simulink model "modelo_XP_LQRY_GUIA"  (R2025b)
settings: Solver=ode4  StartTime=0.0  StopTime=TimeXP  FixedStep=Ts  RelTol=1e-3
values from neighbouring files (symbols this model uses):
  att_alt = 0    [XP_doublets_lqry2.m]    (also in XP_missao_lqry.m; XP_missao_lqry2.m)
  h_ref0 = h_ref    [NL_missao.m]    (also in XP_doublets_lqry2.m = 600; XP_missao.m; XP_missao_lqry.m = XP_h_ref0; XP_missao_lqry2.m = XP_h_ref0)
  phi_psi = XP_dbl_phi_psi    [XP_doublets_lqry2.m]    (also in XP_missao_lqry.m = 0; XP_missao_lqry2.m = cfg_user.phipsi)
  R_accept = cfgm.R    [NL_missao.m]    (also in XP_doublets_lqry2.m = 80; XP_missao.m = XP_R_accept; XP_missao_lqry.m = cfg_user.R; XP_missao_lqry2.m = cfg_user.R)
  refAlt = XP_dbl_refAlt    [XP_doublets_lqry2.m]    (also in XP_missao_lqry.m = 0; XP_missao_lqry2.m = 0)
  refPhi = XP_dbl_refPhi    [XP_doublets_lqry2.m]    (also in XP_missao_lqry.m = 0; XP_missao_lqry2.m = 0)
  refPsi = XP_dbl_refPsi    [XP_doublets_lqry2.m]    (also in XP_missao_lqry.m = 0; XP_missao_lqry2.m = 0)
  reftheta = 0    [XP_doublets_lqry2.m]    (also in XP_missao_lqry.m; XP_missao_lqry2.m)
  refVel = XP_dbl_VT    [XP_doublets_lqry2.m]    (also in XP_missao_lqry.m = 12; XP_missao_lqry2.m = 12)
  VT_ref0 = VT_ref    [NL_missao.m]    (also in XP_doublets_lqry2.m = XP_dbl_VT; XP_missao.m; XP_missao_lqry.m = 12; XP_missao_lqry2.m = 12)
  VT_Throttle = XP_dbl_VT_Throttle    [XP_doublets_lqry2.m]    (also in XP_missao_lqry.m = 1; XP_missao_lqry2.m = 1)
  WPs = WPs_user(1,:)    [NL_missao.m]    (also in XP_doublets_lqry2.m = WPs_user; WPs(:,1:2) = ne'; XP_missao.m; XP_missao_lqry.m; XP_missao_lqry2.m)
  Xe = montaX(y)    [VR_plot_sato_real.m]    (also in VR_tic.m; plot_degrau_3vias_sato.m)
  XP_h_ref0 = XP_msl0    (= 600)    [XP_doublets_lqry2.m]    (also in XP_missao_lqry.m = XP_msl0; XP_missao_lqry2.m = XP_msl0)
  XP_IC_int_alt = double((0 - GsA*[x4_dev; 0]) / GiA)    [XP_doublets_lqry2.m]    (also in XP_missao_lqry.m = (theta0 - GstateLong_Alt*[x4; 0]) / GintLong_Alt; XP_missao_lqry2.m = double((theta0 - GsA*[x4; 0]) / GiA))
  XP_IC_int_speed = double((thr_delta0*100 - GsS*x4_dev) / GiS)    [XP_doublets_lqry2.m]    (also in XP_missao_lqry.m = (XP_thr0*100 - GstateLong_speed*x4) / GintLong_speed; XP_missao_lqry2.m = double((thr_delta0*100 - GsS*x4) / GiS))
  XP_IC_int_theta = double((de_delta0*(1 - GsT(5)) - GsT(1:4)*x4_dev) / GiT)    [XP_doublets_lqry2.m]    (also in XP_missao_lqry.m = (XP_de0_dg*(1 - GstateLong(5)) - GstateLong(1:4)*x4) / GintL; XP_missao_lqry2.m = double((de_delta0*(1 - GsT(5)) - GsT(1:4)*x4) / GiT))
undefined symbols (not defined in the file or in its folder): Gintlat, Gintlat_psi, GintLong, GintLong_Alt, GintLong_speed, GstateLat, GstateLat_psi, GstateLong, GstateLong_Alt, GstateLong_speed
libraries: simulink_extras x14
settings Model: SimulationMode=accelerator  Creator=mirko  LastModifiedBy=kaue

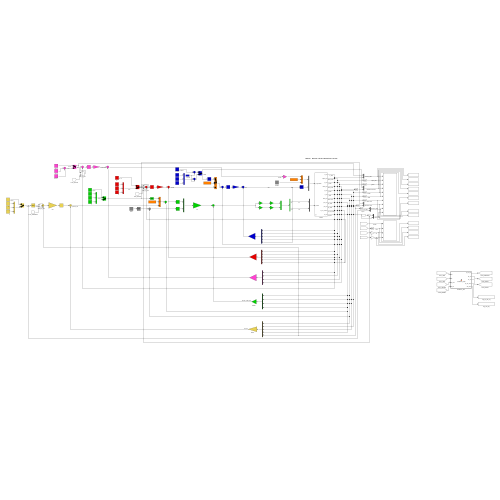
[thumbnail: Simulink's stored preview of the top-level diagram]
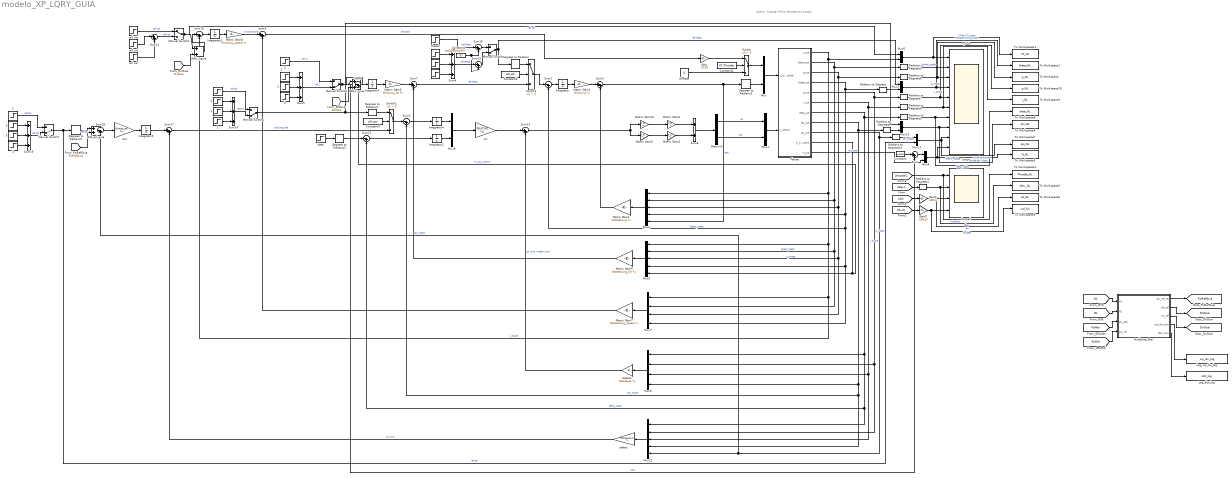
== system modelo_XP_LQRY_GUIA ==
  note: Author: Huascar Mirko Montecinos Cortez
  "   " : Step  Time=80  After=refPhi  SampleTime=0
  "     " : Step  Time=100  After=reftheta  SampleTime=0
  "          " : Step  Time=200  Before=-reftheta  After=0  SampleTime=0
  "            " : Step  Time=150  Before=reftheta  After=-reftheta  SampleTime=0
  "            1" : Step  Time=100  Before=refPhi  After=-refPhi  SampleTime=0
  "            2" : Step  Time=160  Before=refAlt  After=-refAlt  SampleTime=0
  "            3" : Step  Time=100  Before=refPsi  After=-refPsi  SampleTime=0
  "          1" : Step  Time=150  Before=-refPhi  After=0  SampleTime=0
  "          2" : Step  Time=240  Before=-refAlt  After=0  SampleTime=0
  "          3" : Step  Time=150  Before=-refPsi  After=0  SampleTime=0
  "     1" : Step  Time=50  After=refPhi  SampleTime=0
  "     2" : Step  Time=80  After=refAlt  SampleTime=0
  "     3" : Step  Time=50  After=refPsi  SampleTime=0
  "   1" : Step  Time=80  After=refPsi  SampleTime=0
  " Z " : Step  Time=40  After=refAlt  SampleTime=0
  " ref vel " : Step  Time=5  Before=Xe(1)  After=refVel  SampleTime=0
  Add_h_guia : Sum
  Add_psi_guia : Sum
  Add_v_guia : Sum
  Constant : Constant  Value=-Xe(12)
  Constant1 : Constant  Value=rad2deg(Xe(8))
  Constant2 : Constant  Value=VT_Throttle
  Constant3 : Constant  Value=att_alt
  Constant4 : Constant  Value=phi_psi
  Degrees to Radians{,1..3,5} (5 alike) : simulink_extras/Transformations/Degrees to Radians
  Demux4 : Demux  Outputs=2
      settings: DisplayOption=none
  Gain : Gain  Gain=1/100
  Gain1 : Gain  Gain=180/pi
  Gain2 : Gain  Gain=180/pi
  Guidance_Star : MATLAB Function  TreatAsAtomicUnit=on
  Integrator : Integrator  InitialCondition=XP_IC_int_theta
  Integrator1 : Integrator
  Integrator2 : Integrator  InitialCondition=XP_IC_int_alt
  Integrator3 : Integrator  InitialCondition=XP_IC_int_speed
  Integrator4 : Integrator
  Integrator5 : Integrator
  Log_dist_log : ToWorkspace  VariableName=dist_log  SampleTime=-1
  Log_wp_idx_log : ToWorkspace  VariableName=wp_idx_log  SampleTime=-1
  Manual Switch{,2,4,7} (4 alike) : ManualSwitch  CurrentSetting=0
  Manual Switch3 : ManualSwitch
  Matrix Gain1 : Gain  Gain=GstateLong  Multiplication=Matrix(K*u)  SaturateOnIntegerOverflow=on  OutDataTypeStr=Inherit: Same as input  ParamDataTypeStr=Inherit: Same as input
  Matrix Gain10 : Gain  Gain=[1 0]  Multiplication=Matrix(K*u)  SaturateOnIntegerOverflow=on  OutDataTypeStr=Inherit: Same as input  ParamDataTypeStr=Inherit: Same as input
  Matrix Gain2 : Gain  Gain=GintLong  Multiplication=Matrix(K*u)  SaturateOnIntegerOverflow=on  OutDataTypeStr=Inherit: Same as input  ParamDataTypeStr=Inherit: Same as input
  Matrix Gain3 : Gain  Gain=[0 1]'  Multiplication=Matrix(K*u)  SaturateOnIntegerOverflow=on  OutDataTypeStr=Inherit: Same as input  ParamDataTypeStr=Inherit: Same as input
  Matrix Gain4 : Gain  Gain=[1 0]'  Multiplication=Matrix(K*u)  SaturateOnIntegerOverflow=on  OutDataTypeStr=Inherit: Same as input  ParamDataTypeStr=Inherit: Same as input
  Matrix Gain5 : Gain  Gain=GstateLong_Alt  Multiplication=Matrix(K*u)  SaturateOnIntegerOverflow=on  OutDataTypeStr=Inherit: Same as input  ParamDataTypeStr=Inherit: Same as input
  Matrix Gain6 : Gain  Gain=GintLong_Alt  Multiplication=Matrix(K*u)  SaturateOnIntegerOverflow=on  OutDataTypeStr=Inherit: Same as input  ParamDataTypeStr=Inherit: Same as input
  Matrix Gain7 : Gain  Gain=GstateLong_speed  Multiplication=Matrix(K*u)  SaturateOnIntegerOverflow=on  OutDataTypeStr=Inherit: Same as input  ParamDataTypeStr=Inherit: Same as input
  Matrix Gain8 : Gain  Gain=GintLong_speed  Multiplication=Matrix(K*u)  SaturateOnIntegerOverflow=on  OutDataTypeStr=Inherit: Same as input  ParamDataTypeStr=Inherit: Same as input
  Matrix Gain9 : Gain  Gain=[0 1]  Multiplication=Matrix(K*u)  SaturateOnIntegerOverflow=on  OutDataTypeStr=Inherit: Same as input  ParamDataTypeStr=Inherit: Same as input
  Mux{,1,3..4,6,8,10,12} (8 alike) : Mux  Inputs=2
  Mux11 : Mux  Inputs=5
  Mux2 : Mux  Inputs=5
  Mux5 : Mux  Inputs=5
  Mux7 : Mux
  Mux9 : Mux
  Planta : Subsystem
  Radians to Degrees{,1,4..10} (9 alike) : simulink_extras/Transformations/Radians to Degrees
  Scope : Scope  NumInputPorts=10
      settings: ActiveDisplayString=10  ActiveDisplayYMinimum=533.18171177822774  ActiveDisplayYMaximum=1120.7854736880706
  Scope1 : Scope  NumInputPorts=4
      settings: ActiveDisplayString=4  ActiveDisplayYMinimum=-0.044795545594612511  ActiveDisplayYMaximum=0.042922261215851361
  Sum{,3,7,9,11,15..16} (7 alike) : Sum  Inputs=|++
  Sum1 : Sum  Inputs=|-+
  Sum10 : Sum  Inputs=|-+
  Sum12 : Sum  Inputs=|-+  SaturateOnIntegerOverflow=on
  Sum13 : Sum  Inputs=|++  SaturateOnIntegerOverflow=on
  Sum{4..5,14,19} (4 alike) : Sum  Inputs=+++
  Sum17 : Sum  Inputs=|++  SaturateOnIntegerOverflow=on
  Sum18 : Sum  Inputs=|-+  SaturateOnIntegerOverflow=on
  Sum2 : Sum  Inputs=|-+  SaturateOnIntegerOverflow=on
  Sum6 : Sum  Inputs=2  SaturateOnIntegerOverflow=on
  Sum8 : Sum  Inputs=|-+
  Switch : Switch  Criteria=u2 > Threshold  SaturateOnIntegerOverflow=off  InputSameDT=off
  Switch1 : Switch  Criteria=u2 > Threshold  SaturateOnIntegerOverflow=off  InputSameDT=off
  Switch2 : Switch  Criteria=u2 > Threshold  SaturateOnIntegerOverflow=off  InputSameDT=off
  To Workspace : ToWorkspace  VariableName=q_NL  SaveFormat=Structure With Time  SampleTime=-1
  To Workspace1 : ToWorkspace  VariableName=theta_NL  SaveFormat=Structure With Time  SampleTime=-1
  To Workspace10 : ToWorkspace  VariableName=p_NL  SaveFormat=Structure With Time  SampleTime=-1
  To Workspace11 : ToWorkspace  VariableName=VT_NL  SaveFormat=Structure With Time  SampleTime=-1
  To Workspace12 : ToWorkspace  VariableName=Throttle_NL  SaveFormat=Structure With Time  SampleTime=-1
  To Workspace2 : ToWorkspace  VariableName=elev_NL  SaveFormat=Structure With Time  SampleTime=-1
  To Workspace3 : ToWorkspace  VariableName=H_NL  SaveFormat=Structure With Time  SampleTime=-1
  To Workspace4 : ToWorkspace  VariableName=phi_NL  SaveFormat=Structure With Time  SampleTime=-1
  To Workspace5 : ToWorkspace  VariableName=r_NL  SaveFormat=Structure With Time  SampleTime=-1
  To Workspace6 : ToWorkspace  VariableName=ail_NL  SaveFormat=Structure With Time  SampleTime=-1
  To Workspace7 : ToWorkspace  VariableName=psi_NL  SaveFormat=Structure With Time  SampleTime=-1
  To Workspace8 : ToWorkspace  VariableName=beta_NL  SaveFormat=Structure With Time  SampleTime=-1
  To Workspace9 : ToWorkspace  VariableName=rud_NL  SaveFormat=Structure With Time  SampleTime=-1
  beta : Step  Time=0  After=0  SampleTime=0
  int : Gain  Gain=Gintlat  Multiplication=Matrix(K*u)  SaturateOnIntegerOverflow=on  OutDataTypeStr=Inherit: Same as input  ParamDataTypeStr=Inherit: Same as input
  int1 : Gain  Gain=Gintlat_psi  Multiplication=Matrix(K*u)  SaturateOnIntegerOverflow=on  OutDataTypeStr=Inherit: Same as input  ParamDataTypeStr=Inherit: Same as input
  ref vel : Step  Time=15  After=5  SampleTime=0
  "ref vel  " : Step  Time=50  After=-5  SampleTime=0
  states : Gain  Gain=GstateLat_psi  Multiplication=Matrix(K*u)  SaturateOnIntegerOverflow=on  OutDataTypeStr=Inherit: Same as input  ParamDataTypeStr=Inherit: Same as input
  states1 : Gain  Gain=GstateLat  Multiplication=Matrix(K*u)  SaturateOnIntegerOverflow=on  OutDataTypeStr=Inherit: Same as input  ParamDataTypeStr=Inherit: Same as input
  theta2 : Step  Time=100  After=reftheta  SampleTime=0
  throttle : Constant  Value=0
  tag scope: DhGuia=global, DvGuia=global, PsiRefGuia=global
  wires:
  Mux/1 -> Planta/1(u_longitudinal)
  Mux1/1 -> Planta/2(u_lateral)
  Manual Switch/1 -> Degrees to Radians/1, Mux3/1  "ref theta"
  Matrix Gain1/1 -> Sum3/2
  Matrix Gain2/1 -> Sum3/1
  Integrator/1 -> Matrix Gain2/1
  Sum4/1 -> Sum15/1  "ref theta"
  Mux2/1 -> Matrix Gain1/1
  Sum1/1 -> Integrator/1
  Switch1/1 -> Sum1/1
  theta2/1 -> Sum16/1  "ref theta"
  Sum3/1 -> Degrees to Radians3/1, Mux2/5  "elev"
  Planta/1(u_out) -> Mux6/2, Mux7/1, Sum10/2, Mux5/1, Mux2/1  "u_state"
  Planta/2(alpha_out) -> Mux7/2, Mux5/2, Mux2/2, Radians to Degrees5/1  "alpha_state"
  Planta/3(q_out) -> Mux7/3, Mux5/3, Mux2/3, Radians to Degrees6/1  "q_state"
  Planta/4(theta_out) -> Sum1/2, Mux7/4, Mux5/4, Mux2/4, Radians to Degrees/1  "theta_state"
  Planta/5(p_out) -> Radians to Degrees7/1, Mux9/2, Mux11/2  "p_state"
  Planta/6(r_out) -> Radians to Degrees8/1, Mux9/3, Mux11/3  "r_state"
  Planta/7(beta_out) -> Radians to Degrees9/1, Mux11/1, Sum12/2, Mux9/1  "beta_state"
  Planta/8(phi_out) -> Radians to Degrees4/1, Mux11/4, Sum2/2, Mux9/4  "phi_state"
  Planta/9(psi_out) -> Mux11/5, Sum18/2, Radians to Degrees10/1  "psi_state"
  Planta/10(H_out_control) -> Mux5/5, Sum8/2  "H_out_control"
  Mux3/1 -> To Workspace1/1, Scope/4  "thetaref-theta_state"
  Radians to Degrees/1 -> Mux3/2
  Matrix Gain5/1 -> Sum7/2
  " Z "/1 -> Manual Switch2/1  "ref  Z"
  Manual Switch2/1 -> Sum/2, Add_h_guia/1  "ref z"
  Sum8/1 -> Integrator2/1
  Sum7/1 -> Switch1/3  "ref theta"
  Sum5/1 -> Manual Switch2/2  "ref Z"
  Mux5/1 -> Matrix Gain5/1
  Matrix Gain6/1 -> Sum7/1
  Integrator2/1 -> Matrix Gain6/1
  Degrees to Radians/1 -> Switch1/1
  Mux4/1 -> Scope/10, To Workspace3/1  "Href-H_state"
  Constant/1 -> Sum/1
  Sum/1 -> Mux4/1
  Radians to Degrees1/1 -> Scope1/2, To Workspace2/1  "Elev"
  Gain1/1 -> Scope1/3, To Workspace6/1  "Ail"
  Gain2/1 -> Scope1/4, To Workspace9/1  "Rudder"
  "ref vel  "/1 -> Sum11/2
  Sum10/1 -> Integrator3/1
  Mux7/1 -> Matrix Gain7/1
  ref vel/1 -> Sum11/1
  Matrix Gain7/1 -> Sum9/2
  " ref vel "/1 -> Manual Switch3/1  "ref vel"
  Manual Switch3/1 -> Mux6/1, Add_v_guia/1  "ref vel"
  Integrator3/1 -> Matrix Gain8/1
  Sum11/1 -> Manual Switch3/2  "ref vel"
  Matrix Gain8/1 -> Sum9/1  "cmd throttle"
  [Elev] -> Radians to Degrees1/1
  [Ail] -> Gain1/1
  [Rud] -> Gain2/1
  [throttle] -> To Workspace12/1, Scope1/1  "throttle"
  Sum9/1 -> Gain/1  "throttle"
  Mux6/1 -> To Workspace11/1, Scope/1  "VTref-VT_state"
  Matrix Gain9/1 -> Matrix Gain3/1
  Matrix Gain10/1 -> Matrix Gain4/1
  Matrix Gain4/1 -> Sum6/1
  Sum13/1 -> Matrix Gain9/1, Matrix Gain10/1
  Matrix Gain3/1 -> Sum6/2
  Sum6/1 -> Demux4/1
  Demux4/2 -> Mux1/2  "rud"
  Demux4/1 -> Mux1/1  "ail"
  beta/1 -> Degrees to Radians2/1
  "   "/1 -> Manual Switch4/1  "ref phi"
  int/1 -> Sum13/1
  Degrees to Radians2/1 -> Sum12/1
  Mux8/1 -> int/1
  Sum12/1 -> Integrator1/1
  "     1"/1 -> Sum14/1
  Sum14/1 -> Manual Switch4/2  "ref phi"
  "            1"/1 -> Sum14/2
  "          1"/1 -> Sum14/3
  Integrator4/1 -> Mux8/1
  Integrator1/1 -> Mux8/2
  Sum2/1 -> Integrator4/1
  Mux9/1 -> states1/1
  states1/1 -> Sum13/2  "ail cmd, rudder cmd"
  Mux10/1 -> To Workspace4/1, Scope/8  "phiref-phi_state"
  Radians to Degrees4/1 -> Mux10/2
  Manual Switch4/1 -> Mux10/1, Degrees to Radians1/1
  Switch/1 -> Mux/1
  throttle/1 -> Switch/3
  Radians to Degrees5/1 -> Scope/2  "alpha_state"
  Radians to Degrees6/1 -> To Workspace/1, Scope/3  "q_state"
  Radians to Degrees7/1 -> To Workspace10/1, Scope/5  "p_state"
  Radians to Degrees8/1 -> Scope/6, To Workspace5/1  "r_state"
  Radians to Degrees9/1 -> Scope/7, To Workspace8/1  "beta_state"
  Degrees to Radians3/1 -> Mux/2
  Gain/1 -> Switch/1
  Mux12/1 -> To Workspace7/1, Scope/9  "psiref-psi_state"
  Planta/11(H_out) -> Mux4/2  "H_state"
  Constant1/1 -> Sum15/2, Sum16/2
  Sum15/1 -> Manual Switch/2
  Sum16/1 -> Manual Switch/1
  "          "/1 -> Sum4/3
  "     "/1 -> Sum4/1
  "            "/1 -> Sum4/2
  "          2"/1 -> Sum5/3
  "            2"/1 -> Sum5/2
  "     2"/1 -> Sum5/1
  Mux11/1 -> states/1
  Sum18/1 -> int1/1
  Integrator5/1 -> Sum17/1
  Manual Switch7/1 -> Degrees to Radians5/1, Mux12/2  "ref psi"
  int1/1 -> Integrator5/1
  Sum17/1 -> Switch2/3  "psiCmd_rad"
  states/1 -> Sum17/2  "ail cmd"
  Switch2/1 -> Sum2/1
  Degrees to Radians1/1 -> Switch2/1
  "     3"/1 -> Sum19/1
  "            3"/1 -> Sum19/2
  "   1"/1 -> Manual Switch7/1  "ref psi"
  Sum19/1 -> Manual Switch7/2  "ref phi"
  "          3"/1 -> Sum19/3
  Radians to Degrees10/1 -> Mux12/1  "psi_state"
  Constant2/1 -> Switch/2
  Constant3/1 -> Switch1/2
  Constant4/1 -> Switch2/2
  [XN] -> Guidance_Star/1(xN)
  [XE] -> Guidance_Star/2(xE)
  [PsiAbs] -> Guidance_Star/3(psi_abs)
  [PsiRel] -> Guidance_Star/4(psi_rel)
  Guidance_Star/1(psi_ref_rel) -> [PsiRefGuia]
  Guidance_Star/2(dh_ref) -> [DhGuia]
  Guidance_Star/3(dv_ref) -> [DvGuia]
  Guidance_Star/4(wp_idx_mon) -> Log_wp_idx_log/1
  Guidance_Star/5(dist_mon) -> Log_dist_log/1
  Degrees to Radians5/1 -> Add_psi_guia/1  "ref psi"
  [PsiRefGuia] -> Add_psi_guia/2
  Add_psi_guia/1 -> Sum18/1
  [DhGuia] -> Add_h_guia/2
  Add_h_guia/1 -> Sum8/1
  [DvGuia] -> Add_v_guia/2
  Add_v_guia/1 -> Sum10/1

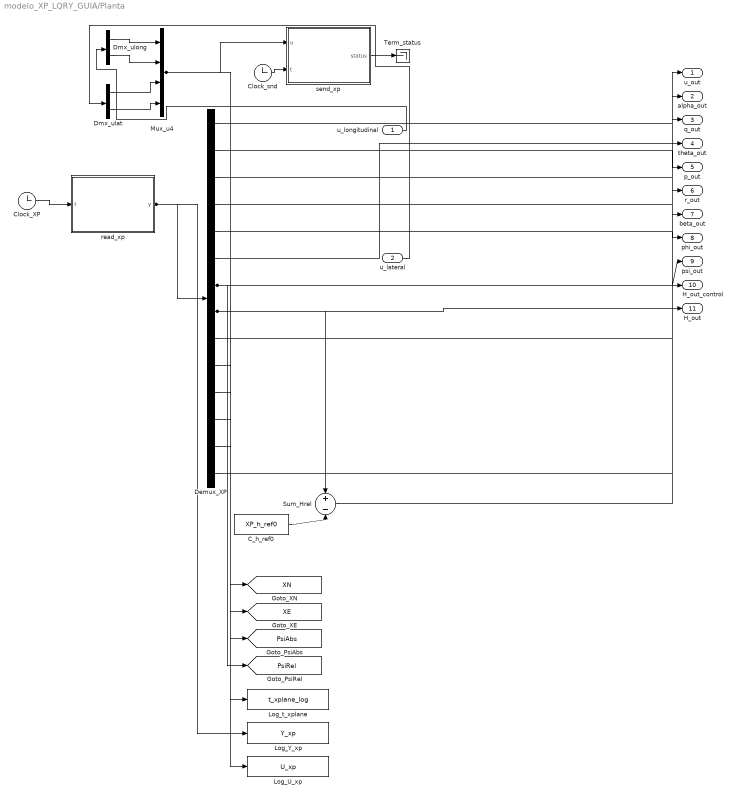
== system modelo_XP_LQRY_GUIA/Planta ==
  u_longitudinal : Inport
  u_lateral : Inport  Port=2
  C_h_ref0 : Constant  Value=XP_h_ref0
  Clock_XP : Clock
  Clock_snd : Clock
  Demux_XP : Demux  Outputs=14
  Dmx_ulat : Demux  Outputs=2
  Dmx_ulong : Demux  Outputs=2
  Log_U_xp : ToWorkspace  VariableName=U_xp  SampleTime=-1
  Log_Y_xp : ToWorkspace  VariableName=Y_xp  SampleTime=-1
  Log_t_xplane : ToWorkspace  VariableName=t_xplane_log  SampleTime=-1
  Mux_u4 : Mux
  Sum_Hrel : Sum  Inputs=+-
  Term_status : Terminator
  read_xp : MATLAB Function  TreatAsAtomicUnit=on
  send_xp : MATLAB Function  TreatAsAtomicUnit=on
  u_out : Outport
  alpha_out : Outport  Port=2
  q_out : Outport  Port=3
  theta_out : Outport  Port=4
  p_out : Outport  Port=5
  r_out : Outport  Port=6
  beta_out : Outport  Port=7
  phi_out : Outport  Port=8
  psi_out : Outport  Port=9
  H_out_control : Outport  Port=10
  H_out : Outport  Port=11
  tag scope: PsiAbs=global, PsiRel=global, XE=global, XN=global
  wires:
  u_longitudinal/1 -> Dmx_ulong/1
  u_lateral/1 -> Dmx_ulat/1
  Dmx_ulong/1 -> Mux_u4/1
  Dmx_ulong/2 -> Mux_u4/2
  Dmx_ulat/1 -> Mux_u4/3
  Dmx_ulat/2 -> Mux_u4/4
  Mux_u4/1 -> send_xp/1(u), Log_U_xp/1
  Clock_snd/1 -> send_xp/2(t)
  send_xp/1(status) -> Term_status/1
  Clock_XP/1 -> read_xp/1(t)
  read_xp/1(y) -> Demux_XP/1, Log_Y_xp/1
  Demux_XP/1 -> u_out/1
  Demux_XP/14 -> alpha_out/1
  Demux_XP/3 -> q_out/1
  Demux_XP/6 -> theta_out/1
  Demux_XP/2 -> p_out/1
  Demux_XP/4 -> r_out/1
  Demux_XP/9 -> beta_out/1
  Demux_XP/5 -> phi_out/1
  Demux_XP/7 -> psi_out/1, [PsiRel]
  Demux_XP/8 -> Sum_Hrel/1, H_out/1
  C_h_ref0/1 -> Sum_Hrel/2
  Sum_Hrel/1 -> H_out_control/1
  Demux_XP/11 -> [XN]
  Demux_XP/12 -> [XE]
  Demux_XP/13 -> [PsiAbs]
  Demux_XP/10 -> Log_t_xplane/1

== matlab function modelo_XP_LQRY_GUIA/Planta/send_xp ==
  settings: updateMethod=DISCRETE  sampleTime=0.05
  data: u input; status output; t input
function status = send_xp(u, t)
%#codegen
coder.extrinsic('xp_send_dh');
persistent k_last
Ts = 0.05;
if isempty(k_last), k_last = -1; end
status = 0;
k_now = floor(t/Ts + 1e-9);
if k_now > k_last
    xp_send_dh(u);
    k_last = k_now;
    status = 1;
end
end

== matlab function modelo_XP_LQRY_GUIA/Planta/read_xp ==
  settings: updateMethod=DISCRETE  sampleTime=0.05
  data: t input; y output
function y = read_xp(t)
%#codegen
coder.extrinsic('xp_read_dh');
persistent y_last k_last
Ts = 0.05;
if isempty(y_last), y_last = zeros(14,1); end
if isempty(k_last), k_last = -1; end
k_now = floor(t/Ts + 1e-9);
y = y_last;
if k_now > k_last
    tmp = zeros(14,1);
    if k_last == -1
        tmp = xp_read_dh(1, t);   % engate: teleporta, reseta psi, ancora pacing
    else
        tmp = xp_read_dh(0, t);   % leitura + pacing de tempo real
    end
    y_last = tmp;
    y = y_last;
    k_last = k_now;
end
end

== matlab function modelo_XP_LQRY_GUIA/Guidance_Star ==
  settings: updateMethod=DISCRETE  sampleTime=0.05
  data: xN input; psi_ref_rel output; xE input; psi_abs input; psi_rel input; dh_ref output; dv_ref output; wp_idx_mon output; dist_mon output; WPs parameter; R_accept parameter; h_ref0 parameter; VT_ref0 parameter
function [psi_ref_rel, dh_ref, dv_ref, wp_idx_mon, dist_mon] = Guidance_Star(xN, xE, psi_abs, psi_rel, WPs, R_accept, h_ref0, VT_ref0)
% Guiagem por waypoints LOS — portado de chart_44 (Guidance_Star) do
% NL_guidance do Julio Machado (PIPER-1-6), adaptado ao harness do DH:
%   - WPs = [Norte(m) Leste(m) Alt MSL(m) Vel(m/s)]; posicao NE relativa
%     ao ENGATE (canais 11-12 do xp_read_dh), LOS em NE absoluto;
%   - wp_idx inicia em 1 (nosso WP1 ja e' o primeiro ALVO; o Julio
%     nascia sobre o WP1 e mirava o 2);
%   - troca de WP: dist <= R_accept && wp_idx < num_wps (segura o ultimo);
%   - psi_los e' proa ABSOLUTA; o harness trabalha com proa RELATIVA ao
%     engate (unwrap continuo, canal 7). Conversao SEM tocar no controle:
%       psi_ref_rel = psi_rel + wrap(psi_los - psi_abs)
%     com wrap(x)=mod(x+pi,2pi)-pi (o calc_erro_proa do Julio) — o erro
%     que chega ao heading hold e' o mesmo, na convencao relativa.
%   - saidas dh_ref/dv_ref sao DELTAS sobre h_ref0/VT_ref0 (as refs de
%     engate do workspace): entram nos pontos dos doublets ja existentes
%     e passam pelos pre-filtros tau_ref do modelo (suavizacao de troca).
persistent wp_idx hold_psi
if isempty(wp_idx), wp_idx = 1; hold_psi = NaN; end
num_wps = size(WPs, 1);
if wp_idx > num_wps, wp_idx = num_wps; end
dist = sqrt((WPs(wp_idx,1) - xN)^2 + (WPs(wp_idx,2) - xE)^2);
if (dist <= R_accept)
    if wp_idx < num_wps
        wp_idx = wp_idx + 1;
    elseif isnan(hold_psi)
        % ADAPTACAO ao DH (difere do Julio, que orbita o ultimo
        % WP): orbitar com LOS puro vira curva continua apertada
        % e o DH nao tem margem de energia p/ isso (G1 2026-08-20:
        % phi 30-50, VT<9). Apos capturar o ULTIMO WP, congela a
        % proa da captura — voo reto nivelado ate o tempo esgotar.
        hold_psi = psi_rel;
    end
end
tN = WPs(wp_idx, 1);
tE = WPs(wp_idx, 2);
psi_los = atan2(tE - xE, tN - xN);
dpsi = mod(psi_los - psi_abs + pi, 2*pi) - pi;
if isnan(hold_psi)
    psi_ref_rel = psi_rel + dpsi;
else
    psi_ref_rel = hold_psi;
end
dh_ref = WPs(wp_idx, 3) - h_ref0;
dv_ref = WPs(wp_idx, 4) - VT_ref0;
wp_idx_mon = wp_idx;
dist_mon = dist;
end
